simulink model "PSB3_0"  (R2021a)
settings: Solver=VariableStepAuto  StartTime=0.0  StopTime=3000  RelTol=1e-3
values from neighbouring files (symbols this model uses):
  n_channel = 1024    [PSB3_0_script.m]    (also in PSB_FPGAdesign8_script.m)
  parallel_factor = 4    [PSB3_0_script.m]    (also in PSB_FPGAdesign8_script.m)
libraries: xbsIndex_r4 x1051, xrbsSSR_Library x154, dspsrcs4 x26
(part 1 of 8)
settings Model: Creator=11037  LastModifiedBy=11037

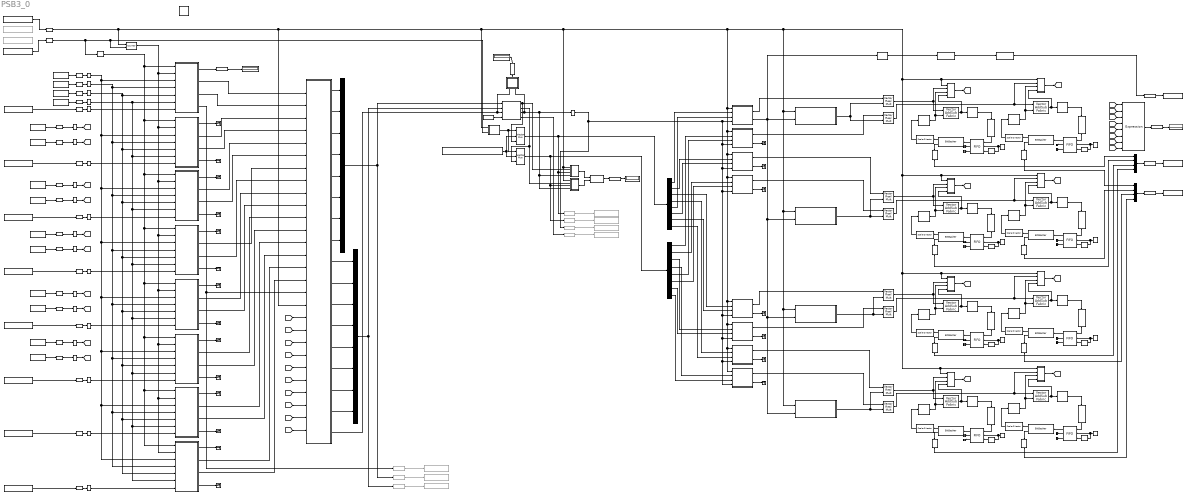
== system PSB3_0 ==
  note: Z^-(10+256)
  note: [zeros(1,50), ones(1,1024), 0]
  note: [zeros(1,50), ones(1,1024), 0]
  note: [zeros(1,50), ones(1,1024), 0]
  note: [zeros(1,50), ones(1,1024), 0]
  note: at t=0, the first samples out of vector FFT are NaN,
  note: With no integer bits at inputs and output, multiply will only saturate for the case of -1 x -1 = 1.
  " System Generator" : xbsIndex_r4/ System Generator  Tag=genX  xilinxfamily=zynquplusRFSOC  part=xczu28dr  speed=-2-e  package=ffvg1517  synthesis_tool=Vivado  clock_wrapper=Clock Enables  directory=C:/PSB3_0_NL  proj_type=Vivado  Synth_file=Vivado Synthesis Defaults  Impl_file=Vivado Implementation Defaults  testbench=off  simulink_period=1  sysclk_period=10  dcm_input_clock_period=10  incr_netlist=off  trim_vbits=Everywhere in SubSystem  dbl_ovrd=According to Block Masks  core_generation=According to Block Masks  run_coregen=off  deprecated_control=off  eval_field=0  block_type=sysgen
  0001_ : Subsystem
  Baseband_even_1 : Subsystem
  Baseband_even_2 : Subsystem
  Baseband_even_3 : Subsystem
  Baseband_even_4 : Subsystem
  Baseband_odd_1 : Subsystem
  Baseband_odd_2 : Subsystem
  Baseband_odd_3 : Subsystem
  Baseband_odd_4 : Subsystem
  BitBasher1 : xbsIndex_r4/BitBasher  bitexpr=|  display_expr=on  sr_1=a  arith_type1=Unsigned  bin_pt1=0  sr_2=b  arith_type2=Unsigned  bin_pt2=0  sr_3=3  arith_type3=Unsigned  bin_pt3=0  sr_4=4  arith_type4=Unsigned  bin_pt4=0  dbl_ovrd=off  block_type=bitbasher
      | a={16'b0, in[255:16]}
      | b={in[15:0]}
  BitBasher2 : xbsIndex_r4/BitBasher  bitexpr=|  display_expr=on  sr_1=a  arith_type1=Unsigned  bin_pt1=0  sr_2=b  arith_type2=Unsigned  bin_pt2=0  sr_3=3  arith_type3=Unsigned  bin_pt3=0  sr_4=4  arith_type4=Unsigned  bin_pt4=0  dbl_ovrd=off  block_type=bitbasher
      | a={16'b0, in[255:16]}
      | b={in[15:0]}
  BitBasher3 : xbsIndex_r4/BitBasher  bitexpr=|  display_expr=on  sr_1=a  arith_type1=Unsigned  bin_pt1=0  sr_2=b  arith_type2=Unsigned  bin_pt2=0  sr_3=3  arith_type3=Unsigned  bin_pt3=0  sr_4=4  arith_type4=Unsigned  bin_pt4=0  dbl_ovrd=off  block_type=bitbasher
      | a={16'b0, in[255:16]}
      | b={in[15:0]}
  BitBasher4 : xbsIndex_r4/BitBasher  bitexpr=|  display_expr=on  sr_1=a  arith_type1=Unsigned  bin_pt1=0  sr_2=b  arith_type2=Unsigned  bin_pt2=0  sr_3=3  arith_type3=Unsigned  bin_pt3=0  sr_4=4  arith_type4=Unsigned  bin_pt4=0  dbl_ovrd=off  block_type=bitbasher
      | a={16'b0, in[255:16]}
      | b={in[15:0]}
  BitBasher5 : xbsIndex_r4/BitBasher  bitexpr=|  display_expr=on  sr_1=a  arith_type1=Unsigned  bin_pt1=0  sr_2=b  arith_type2=Unsigned  bin_pt2=0  sr_3=3  arith_type3=Unsigned  bin_pt3=0  sr_4=4  arith_type4=Unsigned  bin_pt4=0  dbl_ovrd=off  block_type=bitbasher
      | a={16'b0, in[255:16]}
      | b={in[15:0]}
  BitBasher6 : xbsIndex_r4/BitBasher  bitexpr=|  display_expr=on  sr_1=a  arith_type1=Unsigned  bin_pt1=0  sr_2=b  arith_type2=Unsigned  bin_pt2=0  sr_3=3  arith_type3=Unsigned  bin_pt3=0  sr_4=4  arith_type4=Unsigned  bin_pt4=0  dbl_ovrd=off  block_type=bitbasher
      | a={16'b0, in[255:16]}
      | b={in[15:0]}
  BitBasher7 : xbsIndex_r4/BitBasher  bitexpr=|  display_expr=on  sr_1=a  arith_type1=Unsigned  bin_pt1=0  sr_2=b  arith_type2=Unsigned  bin_pt2=0  sr_3=3  arith_type3=Unsigned  bin_pt3=0  sr_4=4  arith_type4=Unsigned  bin_pt4=0  dbl_ovrd=off  block_type=bitbasher
      | a={16'b0, in[255:16]}
      | b={in[15:0]}
  BitBasher8 : xbsIndex_r4/BitBasher  bitexpr=|  display_expr=on  sr_1=a  arith_type1=Unsigned  bin_pt1=0  sr_2=b  arith_type2=Unsigned  bin_pt2=0  sr_3=3  arith_type3=Unsigned  bin_pt3=0  sr_4=4  arith_type4=Unsigned  bin_pt4=0  dbl_ovrd=off  block_type=bitbasher
      | a={16'b0, in[255:16]}
      | b={in[15:0]}
  CORDIC_delay_count_even_1 : Display
  Constant{1..6,14,16} (8 alike) : xbsIndex_r4/Constant  const=1  gui_display_data_type=Boolean  arith_type=Boolean  n_bits=16  bin_pt=14  preci_type=Single  exp_width=8  frac_width=24  explicit_period=on  period=1  equ=P=C  opselect=C  inp2=PCIN>>17  opr=+  inp1=P  carry=CIN  dbl_ovrd=off  block_type=constant
  Constant15 : xbsIndex_r4/Constant  const=2016  gui_display_data_type=Fixed-point  arith_type=Unsigned  n_bits=11  bin_pt=0  preci_type=Single  exp_width=8  frac_width=24  explicit_period=on  period=1  equ=P=C  opselect=C  inp2=PCIN>>17  opr=+  inp1=P  carry=CIN  dbl_ovrd=off  block_type=constant
  DPRAM_FIR_Coeffs_1 : Subsystem
  DPRAM_FIR_Coeffs_2 : Subsystem
  DPRAM_FIR_Coeffs_3 : Subsystem
  DPRAM_FIR_Coeffs_4 : Subsystem
  Delay{1..12,14,16,19,26,31,35,37..38,43..44,48..49} (24 alike) : xbsIndex_r4/Delay  rst=off  infoeditControl=Selection of Reset will increase slice count due to use of real FFs and instead of SRLs  en=off  latency=1  reg_retiming=off  dbl_ovrd=off  block_type=delay
  Delay{13,18,28..30,53,55..56} (8 alike) : xbsIndex_r4/Delay  rst=off  infoeditControl=Selection of Reset will increase slice count due to use of real FFs and instead of SRLs  en=off  latency=1024/parallel_factor-2-1  reg_retiming=off  dbl_ovrd=off  block_type=delay
  Delay15 : xbsIndex_r4/Delay  rst=off  infoeditControl=Selection of Reset will increase slice count due to use of real FFs and instead of SRLs  en=off  latency=2  reg_retiming=off  dbl_ovrd=off  block_type=delay
  Delay17 : xbsIndex_r4/Delay  rst=off  infoeditControl=Selection of Reset will increase slice count due to use of real FFs and instead of SRLs  en=off  latency=5  reg_retiming=off  dbl_ovrd=off  block_type=delay
  Delay54 : xbsIndex_r4/Delay  rst=off  infoeditControl=Selection of Reset will increase slice count due to use of real FFs and instead of SRLs  en=off  latency=1024/parallel_factor  reg_retiming=off  dbl_ovrd=off  block_type=delay
  Delay_duration : Display
  Demux : Demux  Outputs=8
  Demux1 : Demux  Outputs=8
  Display ov_add : Display
      settings: Format=decimal (Stored Integer)
  Expression : xbsIndex_r4/Expression  expression=a | b  align_bp=off  en=off  latency=1  precision=Full  arith_type=Unsigned  n_bits=1  bin_pt=0  dbl_ovrd=off  block_type=expr
  Expression1 : xbsIndex_r4/Expression  expression=a1 | b1 | c1 | d1 | a2 | b2 | c2 | d2  align_bp=off  en=off  latency=1  precision=Full  arith_type=Unsigned  n_bits=1  bin_pt=0  dbl_ovrd=off  block_type=expr
  FIFO{1..8} (8 alike) : xbsIndex_r4/FIFO  mem_type=Block RAM  performance_options=Standard_FIFO  embedded_registers=off  depth=1K  percent_nbits=1  rst=off  rst_latency=2  en=off  use_dcount=off  use_percent_full_port=off  use_almost_empty=off  almost_empty_thresh=2  use_almost_full=off  use_rd_rst_busy=off  use_wr_rst_busy=off  almost_full_thresh=14  explicit_period=off  dbl_ovrd=off  simulation_type=fast_sim  block_type=fifo
  Gin_TL_reset : xbsIndex_r4/Gateway In  gui_display_data_type=Boolean  arith_type=Boolean  n_bits=18  bin_pt=15  preci_type=Single  exp_width=8  frac_width=24  rows=1  columns=1  quantization="Round  (unbiased: +/- Inf)"  overflow=Flag as error  period=1  UseAsADC=off  ADCChannel='1'  interface=None  automatic_assignment=on  address_offset=hex2dec('00')  intf_name=''  intf_description=''  default_value=0  timing_constraint=None  locs_specified=off  LOCs={}  io_standard={}  inherit_from_input=off  hdl_port=on  dbl_ovrd=off  block_type=gatewayin
  Gin_TL_start : xbsIndex_r4/Gateway In  gui_display_data_type=Boolean  arith_type=Boolean  n_bits=18  bin_pt=15  preci_type=Single  exp_width=8  frac_width=24  rows=1  columns=1  quantization="Round  (unbiased: +/- Inf)"  overflow=Flag as error  period=1  UseAsADC=off  ADCChannel='1'  interface=None  automatic_assignment=on  address_offset=hex2dec('00')  intf_name=''  intf_description=''  default_value=0  timing_constraint=None  locs_specified=off  LOCs={}  io_standard={}  inherit_from_input=off  hdl_port=on  dbl_ovrd=off  block_type=gatewayin
  Gin_addr : xbsIndex_r4/Gateway In  gui_display_data_type=Fixed-point  arith_type=Unsigned  n_bits=10-2  bin_pt=0  preci_type=Single  exp_width=8  frac_width=24  rows=1  columns=1  quantization=Truncate  overflow=Flag as error  period=1  UseAsADC=off  ADCChannel='1'  interface=None  automatic_assignment=on  address_offset=hex2dec('00')  intf_name=''  intf_description=''  default_value=0  timing_constraint=None  locs_specified=off  LOCs={}  io_standard={}  inherit_from_input=off  hdl_port=on  dbl_ovrd=off  block_type=gatewayin
  Gin_dphi : xbsIndex_r4/Gateway In  gui_display_data_type=Fixed-point  arith_type=Unsigned  n_bits=16  bin_pt=0  preci_type=Single  exp_width=8  frac_width=24  rows=1  columns=1  quantization=Truncate  overflow=Flag as error  period=1  UseAsADC=off  ADCChannel='1'  interface=None  automatic_assignment=on  address_offset=hex2dec('00')  intf_name=''  intf_description=''  default_value=0  timing_constraint=None  locs_specified=off  LOCs={}  io_standard={}  inherit_from_input=off  hdl_port=on  dbl_ovrd=off  block_type=gatewayin
  Gin_init_im : xbsIndex_r4/Gateway In  gui_display_data_type=Fixed-point  arith_type="Signed  (2's comp)"  n_bits=18  bin_pt=16  preci_type=Single  exp_width=8  frac_width=24  rows=1  columns=1  quantization=Truncate  overflow=Flag as error  period=1  UseAsADC=off  ADCChannel='1'  interface=None  automatic_assignment=on  address_offset=hex2dec('00')  intf_name=''  intf_description=''  default_value=0  timing_constraint=None  locs_specified=off  LOCs={}  io_standard={}  inherit_from_input=off  hdl_port=on  dbl_ovrd=off  block_type=gatewayin
  Gin_init_re : xbsIndex_r4/Gateway In  gui_display_data_type=Fixed-point  arith_type="Signed  (2's comp)"  n_bits=18  bin_pt=16  preci_type=Single  exp_width=8  frac_width=24  rows=1  columns=1  quantization=Truncate  overflow=Flag as error  period=1  UseAsADC=off  ADCChannel='1'  interface=None  automatic_assignment=on  address_offset=hex2dec('00')  intf_name=''  intf_description=''  default_value=0  timing_constraint=None  locs_specified=off  LOCs={}  io_standard={}  inherit_from_input=off  hdl_port=on  dbl_ovrd=off  block_type=gatewayin
  Gin_we_even_{1..4} (4 alike) : xbsIndex_r4/Gateway In  gui_display_data_type=Boolean  arith_type=Boolean  n_bits=18  bin_pt=15  preci_type=Single  exp_width=8  frac_width=24  rows=1  columns=1  quantization="Round  (unbiased: +/- Inf)"  overflow=Flag as error  period=1  UseAsADC=off  ADCChannel='1'  interface=None  automatic_assignment=on  address_offset=hex2dec('00')  intf_name=''  intf_description=''  default_value=0  timing_constraint=None  locs_specified=off  LOCs={}  io_standard={}  inherit_from_input=off  hdl_port=on  dbl_ovrd=off  block_type=gatewayin
  Gin_we_odd_{1..4} (4 alike) : xbsIndex_r4/Gateway In  gui_display_data_type=Boolean  arith_type=Boolean  n_bits=18  bin_pt=15  preci_type=Single  exp_width=8  frac_width=24  rows=1  columns=1  quantization="Round  (unbiased: +/- Inf)"  overflow=Flag as error  period=1  UseAsADC=off  ADCChannel='1'  interface=None  automatic_assignment=on  address_offset=hex2dec('00')  intf_name=''  intf_description=''  default_value=0  timing_constraint=None  locs_specified=off  LOCs={}  io_standard={}  inherit_from_input=off  hdl_port=on  dbl_ovrd=off  block_type=gatewayin
  Gout_CORDIC_delay_even_1 : xbsIndex_r4/Gateway Out  inherit_from_input=on  hdl_port=on  rows=1  columns=1  UseAsDAC=off  DACChannel='1'  interface=None  automatic_assignment=on  address_offset=hex2dec('00')  intf_name=''  intf_description=''  timing_constraint=None  locs_specified=off  LOCs={}  io_standard={}  block_type=gatewayout
  Gout_CORDIC_im : xrbsSSR_Library/Vector Real Gateway Out  Commented=on  inherit_from_input=off  hdl_port=on  rows=1  columns=1  UseAsDAC=off  DACChannel='1'  interface=None  automatic_assignment=on  address_offset=hex2dec('00')  intf_name=''  intf_description=''  timing_constraint=None  locs_specified=off  LOCs={}  io_standard={}  block_type=realgatewayout_ssr  sg_ssr=8  sg_ssr_prev=8  sg_ssr_name=vect_real_gwayout
      settings: SourceProductName=Xilinx SSR Blockset  infoedit=The Vector Real Gateway out block converts Xilinx fixed-point or floating-point type vector inputs into vector ouputs of type Simulink integer, single, double, or fixed-point.<br><br>Hardware notes: In hardware these blocks become top level output ports or are discarded, depending on how they are configured.
  Gout_CORDIC_re : xrbsSSR_Library/Vector Real Gateway Out  Commented=on  inherit_from_input=on  hdl_port=on  rows=1  columns=1  UseAsDAC=off  DACChannel='1'  interface=None  automatic_assignment=on  address_offset=hex2dec('00')  intf_name=''  intf_description=''  timing_constraint=None  locs_specified=off  LOCs={}  io_standard={}  block_type=realgatewayout_ssr  sg_ssr=8  sg_ssr_prev=8  sg_ssr_name=vect_real_gwayout
      settings: SourceProductName=Xilinx SSR Blockset  infoedit=The Vector Real Gateway out block converts Xilinx fixed-point or floating-point type vector inputs into vector ouputs of type Simulink integer, single, double, or fixed-point.<br><br>Hardware notes: In hardware these blocks become top level output ports or are discarded, depending on how they are configured.
  Gout_CORDIC_tvalid : xbsIndex_r4/Gateway Out  Commented=on  inherit_from_input=on  hdl_port=on  rows=1  columns=1  UseAsDAC=off  DACChannel='1'  interface=None  automatic_assignment=on  address_offset=hex2dec('00')  intf_name=''  intf_description=''  timing_constraint=None  locs_specified=off  LOCs={}  io_standard={}  block_type=gatewayout
  Gout_PSB_im : xrbsSSR_Library/Vector Real Gateway Out  inherit_from_input=on  hdl_port=on  rows=1  columns=1  UseAsDAC=off  DACChannel='1'  interface=None  automatic_assignment=on  address_offset=hex2dec('00')  intf_name=''  intf_description=''  timing_constraint=None  locs_specified=off  LOCs={}  io_standard={}  block_type=realgatewayout_ssr  sg_ssr=4  sg_ssr_prev=4  sg_ssr_name=vect_real_gwayout
      settings: SourceProductName=Xilinx SSR Blockset  infoedit=The Vector Real Gateway out block converts Xilinx fixed-point or floating-point type vector inputs into vector ouputs of type Simulink integer, single, double, or fixed-point.<br><br>Hardware notes: In hardware these blocks become top level output ports or are discarded, depending on how they are configured.
  Gout_PSB_re : xrbsSSR_Library/Vector Real Gateway Out  inherit_from_input=on  hdl_port=on  rows=1  columns=1  UseAsDAC=off  DACChannel='1'  interface=None  automatic_assignment=on  address_offset=hex2dec('00')  intf_name=''  intf_description=''  timing_constraint=None  locs_specified=off  LOCs={}  io_standard={}  block_type=realgatewayout_ssr  sg_ssr=4  sg_ssr_prev=4  sg_ssr_name=vect_real_gwayout
      settings: SourceProductName=Xilinx SSR Blockset  infoedit=The Vector Real Gateway out block converts Xilinx fixed-point or floating-point type vector inputs into vector ouputs of type Simulink integer, single, double, or fixed-point.<br><br>Hardware notes: In hardware these blocks become top level output ports or are discarded, depending on how they are configured.
  Gout_PSB_tvalid : xbsIndex_r4/Gateway Out  inherit_from_input=on  hdl_port=on  rows=1  columns=1  UseAsDAC=off  DACChannel='1'  interface=None  automatic_assignment=on  address_offset=hex2dec('00')  intf_name=''  intf_description=''  timing_constraint=None  locs_specified=off  LOCs={}  io_standard={}  block_type=gatewayout
  Gout_delay_iFFT : xbsIndex_r4/Gateway Out  inherit_from_input=on  hdl_port=on  rows=1  columns=1  UseAsDAC=off  DACChannel='1'  interface=None  automatic_assignment=on  address_offset=hex2dec('00')  intf_name=''  intf_description=''  timing_constraint=None  locs_specified=off  LOCs={}  io_standard={}  block_type=gatewayout
  Gout_ov_IFFT : xbsIndex_r4/Gateway Out  inherit_from_input=on  hdl_port=on  rows=1  columns=1  UseAsDAC=off  DACChannel='1'  interface=None  automatic_assignment=on  address_offset=hex2dec('00')  intf_name=''  intf_description=''  timing_constraint=None  locs_specified=off  LOCs={}  io_standard={}  block_type=gatewayout
  Gout_ov_add : xbsIndex_r4/Gateway Out  inherit_from_input=on  hdl_port=on  rows=1  columns=1  UseAsDAC=off  DACChannel='1'  interface=None  automatic_assignment=on  address_offset=hex2dec('00')  intf_name=''  intf_description=''  timing_constraint=None  locs_specified=off  LOCs={}  io_standard={}  block_type=gatewayout
  Gout_vIFFT_im : xrbsSSR_Library/Vector Real Gateway Out  Commented=on  inherit_from_input=off  hdl_port=on  rows=1  columns=1  UseAsDAC=off  DACChannel='1'  interface=None  automatic_assignment=on  address_offset=hex2dec('00')  intf_name=''  intf_description=''  timing_constraint=None  locs_specified=off  LOCs={}  io_standard={}  block_type=realgatewayout_ssr  sg_ssr=8  sg_ssr_prev=8  sg_ssr_name=vect_real_gwayout
      settings: SourceProductName=Xilinx SSR Blockset  infoedit=The Vector Real Gateway out block converts Xilinx fixed-point or floating-point type vector inputs into vector ouputs of type Simulink integer, single, double, or fixed-point.<br><br>Hardware notes: In hardware these blocks become top level output ports or are discarded, depending on how they are configured.
  Gout_vIFFT_re : xrbsSSR_Library/Vector Real Gateway Out  Commented=on  inherit_from_input=off  hdl_port=on  rows=1  columns=1  UseAsDAC=off  DACChannel='1'  interface=None  automatic_assignment=on  address_offset=hex2dec('00')  intf_name=''  intf_description=''  timing_constraint=None  locs_specified=off  LOCs={}  io_standard={}  block_type=realgatewayout_ssr  sg_ssr=8  sg_ssr_prev=8  sg_ssr_name=vect_real_gwayout
      settings: SourceProductName=Xilinx SSR Blockset  infoedit=The Vector Real Gateway out block converts Xilinx fixed-point or floating-point type vector inputs into vector ouputs of type Simulink integer, single, double, or fixed-point.<br><br>Hardware notes: In hardware these blocks become top level output ports or are discarded, depending on how they are configured.
  Gout_vIFFT_scale : xbsIndex_r4/Gateway Out  Commented=on  inherit_from_input=on  hdl_port=on  rows=1  columns=1  UseAsDAC=off  DACChannel='1'  interface=None  automatic_assignment=on  address_offset=hex2dec('00')  intf_name=''  intf_description=''  timing_constraint=None  locs_specified=off  LOCs={}  io_standard={}  block_type=gatewayout
  Gout_vIFFT_tvalid : xbsIndex_r4/Gateway Out  Commented=on  inherit_from_input=off  hdl_port=on  rows=1  columns=1  UseAsDAC=off  DACChannel='1'  interface=None  automatic_assignment=on  address_offset=hex2dec('00')  intf_name=''  intf_description=''  timing_constraint=None  locs_specified=off  LOCs={}  io_standard={}  block_type=gatewayout
  Mux : Mux  Inputs=8
  Mux1 : Mux  Inputs=8
  Mux2 : Mux
  Mux3 : Mux
  Overflow Detector add_im_1 : Subsystem
  Overflow Detector add_im_2 : Subsystem
  Overflow Detector add_im_3 : Subsystem
  Overflow Detector add_im_4 : Subsystem
  Overflow Detector add_re_1 : Subsystem
  Overflow Detector add_re_2 : Subsystem
  Overflow Detector add_re_3 : Subsystem
  Overflow Detector add_re_4 : Subsystem
  RAM_dphi_addr : xbsIndex_r4/Counter  cnt_type=Free Running  cnt_to=Inf  operation=Up  start_count=0  cnt_by_val=1  arith_type=Unsigned  n_bits=10-2  bin_pt=0  load_pin=off  rst=on  en=on  explicit_period=on  period=1  use_behavioral_HDL=off  implementation=DSP48  dbl_ovrd=off  block_type=counter
  Reinterpret{,1..7} (8 alike) : xbsIndex_r4/Reinterpret  force_arith_type=on  arith_type="Signed  (2's comp)"  force_bin_pt=on  bin_pt=14  block_type=reinterpret
  Scalar to Vector{1..8} (8 alike) : xrbsSSR_Library/Scalar2Vector  Width=16  sg_ssr=16  sg_ssr_prev=16  sg_ssr_name=vect_Scalar2Vector  block_type=scalar2vector_ssr
      settings: SourceProductName=Xilinx SSR Blockset
  TL_reset : dspsrcs4/Signal From Workspace  Commented=on  X="[zeros(1,1000), ones(1,3000),  0]"  Ts=1  nsamps=1  OutputAfterFinalValue=Holding final value  ignoreOrWarnInputAndFrameLengths=on  OutputFrames=off
  TL_reset1 : dspsrcs4/Signal From Workspace  X=0  Ts=1  nsamps=1  OutputAfterFinalValue=Holding final value  ignoreOrWarnInputAndFrameLengths=on  OutputFrames=off
  TL_start : dspsrcs4/Signal From Workspace  Commented=on  X=[ones(1,1000), zeros(1,3000), 1]  Ts=1  nsamps=1  OutputAfterFinalValue=Holding final value  ignoreOrWarnInputAndFrameLengths=on  OutputFrames=off
  TL_start1 : dspsrcs4/Signal From Workspace  X=1  Ts=1  nsamps=1  OutputAfterFinalValue=Holding final value  ignoreOrWarnInputAndFrameLengths=on  OutputFrames=off
  TS_{0..7} (8 alike) : xbsIndex_r4/Gateway In  gui_display_data_type=Fixed-point  arith_type=Unsigned  n_bits=12  bin_pt=0  preci_type=Single  exp_width=8  frac_width=24  rows=1  columns=1  quantization=Truncate  overflow=Flag as error  period=1  UseAsADC=off  ADCChannel='1'  interface=None  automatic_assignment=on  address_offset=hex2dec('00')  intf_name=''  intf_description=''  default_value=0  timing_constraint=None  locs_specified=off  LOCs={}  io_standard={}  inherit_from_input=off  hdl_port=on  dbl_ovrd=off  block_type=gatewayin
  TS_A : xbsIndex_r4/Gateway In  gui_display_data_type=Fixed-point  arith_type=Unsigned  n_bits=8  bin_pt=0  preci_type=Single  exp_width=8  frac_width=24  rows=1  columns=1  quantization=Truncate  overflow=Flag as error  period=1  UseAsADC=off  ADCChannel='1'  interface=None  automatic_assignment=on  address_offset=hex2dec('00')  intf_name=''  intf_description=''  default_value=0  timing_constraint=None  locs_specified=off  LOCs={}  io_standard={}  inherit_from_input=off  hdl_port=on  dbl_ovrd=off  block_type=gatewayin
  TS_W : xbsIndex_r4/Gateway In  gui_display_data_type=Boolean  arith_type=Boolean  n_bits=18  bin_pt=15  preci_type=Single  exp_width=8  frac_width=24  rows=1  columns=1  quantization="Round  (unbiased: +/- Inf)"  overflow=Flag as error  period=1  UseAsADC=off  ADCChannel='1'  interface=None  automatic_assignment=on  address_offset=hex2dec('00')  intf_name=''  intf_description=''  default_value=0  timing_constraint=None  locs_specified=off  LOCs={}  io_standard={}  inherit_from_input=off  hdl_port=on  dbl_ovrd=off  block_type=gatewayin
  Terminator{,1..36} (37 alike) : Terminator
  To Workspace1 : ToWorkspace  Commented=on  VariableName=vIFFT_out_scale  SampleTime=1
  To Workspace10 : ToWorkspace  VariableName=PSB_out_im  SampleTime=1
  To Workspace2 : ToWorkspace  Commented=on  VariableName=vIFFT_out_re  SampleTime=1
  To Workspace3 : ToWorkspace  Commented=on  VariableName=vIFFT_out_im  SampleTime=1
  To Workspace4 : ToWorkspace  Commented=on  VariableName=CORDIC_out_re  SampleTime=1
  To Workspace5 : ToWorkspace  Commented=on  VariableName=vIFFT_out_tvalid  SampleTime=1
  To Workspace6 : ToWorkspace  VariableName=PSB_out_tvalid  SampleTime=1
  To Workspace7 : ToWorkspace  VariableName=PSB_out_re  SampleTime=1
  To Workspace8 : ToWorkspace  Commented=on  VariableName=CORDIC_out_im  SampleTime=1
  To Workspace9 : ToWorkspace  Commented=on  VariableName=CORDIC_out_tvalid  SampleTime=1
  ToneSelect : Subsystem
  Vector AddSub Fabric{,1..7} (8 alike) : xrbsSSR_Library/Vector AddSub Fabric  mode=Addition  use_carryin=off  use_carryout=off  en=off  sg_latency=2  precision=User Defined  arith_type="Signed  (2's comp)"  n_bits=16  bin_pt=14  quantization=Truncate  overflow=Flag as error  use_behavioral_HDL=off  hw_selection=DSP48  pipelined=off  dbl_ovrd=off  block_type=addsub_ssr  sg_ssr=16  sg_ssr_prev=16  sg_ssr_name=vect_addsubfab
      settings: SourceProductName=Xilinx SSR Blockset
  Vector Constant : xrbsSSR_Library/Vector Constant  const=[0.9 0.9 0.9 0.9 0.9 0.9 0.9 0.9]  gui_display_data_type=Fixed-point  arith_type=Signed (2's comp)  n_bits=16  bin_pt=15  preci_type=Single  exp_width=8  frac_width=24  explicit_period=on  period=1  sg_ssr=8  sg_ssr_prev=8  equ=P=C  opselect=C  inp2=PCIN>>17  opr=+  inp1=P  carry=CIN  dbl_ovrd=off  block_type=constant_ssr
      settings: SourceProductName=Xilinx SSR Blockset
  Vector Mux : xrbsSSR_Library/Vector Mux  inputs=2  inputs_prev=2  en=off  vectorize_en=off  vectorize_sel=off  sg_latency=1  precision=User Defined  arith_type="Signed  (2's comp)"  n_bits=16  bin_pt=15  quantization=Truncate  overflow=Saturate  dbl_ovrd=off  block_type=mux_ssr  sg_ssr=8  sg_ssr_prev=8  sg_ssr_name=vect_mux
      settings: SourceProductName=Xilinx SSR Blockset  infoedit=The Vector Multiplexer block supports Multiplexing feature for input of vector types.
  Vector Mux1 : xrbsSSR_Library/Vector Mux  inputs=2  inputs_prev=2  en=off  vectorize_en=off  vectorize_sel=off  sg_latency=1  precision=User Defined  arith_type="Signed  (2's comp)"  n_bits=16  bin_pt=15  quantization=Truncate  overflow=Saturate  dbl_ovrd=off  block_type=mux_ssr  sg_ssr=8  sg_ssr_prev=8  sg_ssr_name=vect_mux
      settings: SourceProductName=Xilinx SSR Blockset  infoedit=The Vector Multiplexer block supports Multiplexing feature for input of vector types.
  Vector Real Mult Im_{1..4} (4 alike) : xrbsSSR_Library/Vector Real Mult  sg_ssr=16  sg_ssr_prev=16  precision=User Defined  arith_type="Signed  (2's comp)"  n_bits=16  bin_pt=15  quantization=Truncate  overflow=Saturate  en=off  sg_latency=5  use_behavioral_HDL=off  opt=Speed  use_embedded=on  optimum_pipeline=off  pipeline=on  dbl_ovrd=off  use_rpm=on  placement_style=Triangular  block_type=realmult_ssr  sg_ssr_name=vect_realmult
      settings: SourceProductName=Xilinx SSR Blockset  infoedit=The Vector Real Multiplier block supports multiplicatoin feature for vector input types.<br><br>Hardware notes: To check for the optimum internal pipeline stages of the dedicated multiplier you must select 'Test for optimum pipelining'.<br><br>Optimization Goal: For implementation into device fabric(LUTs),the Speed and Area optimization will take effect only it its supported by IP for the particular device family. Otherwise, the results will be identical regardless of the selection.
  Vector Real Mult Re_{1..4} (4 alike) : xrbsSSR_Library/Vector Real Mult  sg_ssr=16  sg_ssr_prev=16  precision=User Defined  arith_type="Signed  (2's comp)"  n_bits=16  bin_pt=15  quantization=Truncate  overflow=Saturate  en=off  sg_latency=5  use_behavioral_HDL=off  opt=Speed  use_embedded=on  optimum_pipeline=off  pipeline=on  dbl_ovrd=off  use_rpm=on  placement_style=Triangular  block_type=realmult_ssr  sg_ssr_name=vect_realmult
      settings: SourceProductName=Xilinx SSR Blockset  infoedit=The Vector Real Multiplier block supports multiplicatoin feature for vector input types.<br><br>Hardware notes: To check for the optimum internal pipeline stages of the dedicated multiplier you must select 'Test for optimum pipelining'.<br><br>Optimization Goal: For implementation into device fabric(LUTs),the Speed and Area optimization will take effect only it its supported by IP for the particular device family. Otherwise, the results will be identical regardless of the selection.
  Vector Reinterpret{1..3,6,9..11,14} (8 alike) : xrbsSSR_Library/Vector Reinterpret  sg_ssr=16  sg_ssr_prev=16  force_arith_type=on  arith_type="Signed  (2's comp)"  force_bin_pt=on  bin_pt=14  block_type=reinterpret_ssr
      settings: SourceProductName=Xilinx SSR Blockset  infoedit="The Vector Reinterpret block Changes vector input signal type without altering the binary representation. You can change the signal between signed and unsigned, and relocate the binary point.<br><br>Hardware notes: In hardware this block costs nothing.<br><br>Example:  Suppose the input is 6 bits wide, signed, with 2 fractional bits, and the output is forced to unsigned with 0 fractional bits.  Then an input of -2.0 (1110.00 in binary 2's complement) becomes an output of 56 (111000 in binary)."
  Vector Reinterpret{4..5,7..8,12..13,15..16} (8 alike) : xrbsSSR_Library/Vector Reinterpret  sg_ssr=16  sg_ssr_prev=16  force_arith_type=on  arith_type=Unsigned  force_bin_pt=on  bin_pt=0  block_type=reinterpret_ssr
      settings: SourceProductName=Xilinx SSR Blockset  infoedit="The Vector Reinterpret block Changes vector input signal type without altering the binary representation. You can change the signal between signed and unsigned, and relocate the binary point.<br><br>Hardware notes: In hardware this block costs nothing.<br><br>Example:  Suppose the input is 6 bits wide, signed, with 2 fractional bits, and the output is forced to unsigned with 0 fractional bits.  Then an input of -2.0 (1110.00 in binary 2's complement) becomes an output of 56 (111000 in binary)."
  Vector to Scalar{,1..7} (8 alike) : xrbsSSR_Library/Vector2Scalar  sg_ssr=16  sg_ssr_prev=16  sg_ssr_name=vect_Vector2Scalar  block_type=vector2scalar_ssr
      settings: SourceProductName=Xilinx SSR Blockset
  delayCounter : Subsystem
  ov_IFFT Display : Display
      settings: Format=decimal (Stored Integer)
  ov_detector_IFFT_im : Subsystem
  ov_detector_IFFT_re : Subsystem
  reordering extending buffer imag_1 : Subsystem
  reordering extending buffer imag_2 : Subsystem
  reordering extending buffer imag_3 : Subsystem
  reordering extending buffer imag_4 : Subsystem
  reordering extending buffer real_1 : Subsystem
  reordering extending buffer real_2 : Subsystem
  reordering extending buffer real_3 : Subsystem
  reordering extending buffer real_4 : Subsystem
  test_TS_{0..7} (8 alike) : dspsrcs4/Signal From Workspace  X=0  Ts=1  nsamps=1  OutputAfterFinalValue=Setting to zero  ignoreOrWarnInputAndFrameLengths=on  OutputFrames=off
  test_TS_A : dspsrcs4/Signal From Workspace  X=0  Ts=1  nsamps=1  OutputAfterFinalValue=Setting to zero  ignoreOrWarnInputAndFrameLengths=on  OutputFrames=off
  test_TS_W : dspsrcs4/Signal From Workspace  X=0  Ts=1  nsamps=1  OutputAfterFinalValue=Setting to zero  ignoreOrWarnInputAndFrameLengths=on  OutputFrames=off
  vector IFFT : Subsystem
  w_addr : dspsrcs4/Signal From Workspace  X=[0:255]  Ts=1  nsamps=1  OutputAfterFinalValue=Setting to zero  ignoreOrWarnInputAndFrameLengths=on  OutputFrames=off
  w_dphi : dspsrcs4/Signal From Workspace  X=dphi_uint16_odd_4  Ts=1  nsamps=1  OutputAfterFinalValue=Setting to zero  ignoreOrWarnInputAndFrameLengths=on  OutputFrames=off
  w_init_im : dspsrcs4/Signal From Workspace  X=init_im_odd_4  Ts=1  nsamps=1  OutputAfterFinalValue=Setting to zero  ignoreOrWarnInputAndFrameLengths=on  OutputFrames=off
  w_init_re : dspsrcs4/Signal From Workspace  X=init_re_odd_4  Ts=1  nsamps=1  OutputAfterFinalValue=Setting to zero  ignoreOrWarnInputAndFrameLengths=on  OutputFrames=off
  we_even_{1..4} (4 alike) : dspsrcs4/Signal From Workspace  X=[0]  Ts=1  nsamps=1  OutputAfterFinalValue=Holding final value  ignoreOrWarnInputAndFrameLengths=on  OutputFrames=off
  we_odd_{1..4} (4 alike) : dspsrcs4/Signal From Workspace  X=[0]  Ts=1  nsamps=1  OutputAfterFinalValue=Holding final value  ignoreOrWarnInputAndFrameLengths=on  OutputFrames=off
  wires:
  Delay1/1 -> Baseband_even_1/7(we)
  Reinterpret2/1 -> Mux3/2
  Delay37/1 -> Baseband_even_1/6(dphi_even), Baseband_odd_1/6(dphi_odd), Baseband_even_2/6(dphi_even_2), Baseband_odd_2/6(dphi_odd_2), Baseband_even_3/6(dphi_even), Baseband_odd_3/6(dphi_odd), Baseband_even_4/6(dphi_even_2), Baseband_odd_4/6(dphi_odd_2)
  Constant16/1 -> Delay18/1, FIFO3/2
  Vector Real Mult Re_3/1 -> Overflow Detector add_re_3/2(A), Vector AddSub Fabric4/1
  reordering extending buffer real_4/2(out_tvalid) -> Terminator28/1
  Baseband_odd_3/4(out_tvalid) -> Terminator10/1
  0001_/1(out) -> Vector Mux1/1, Vector Mux/1
  Gout_vIFFT_tvalid/1 -> To Workspace5/1  "op_valid"
  we_odd_2/1 -> Gin_we_odd_2/1  "we"
  Reinterpret5/1 -> Mux2/4
  w_init_re/1 -> Gin_init_re/1
  Gin_TL_reset/1 -> ToneSelect/18(rst), ov_detector_IFFT_im/1(rst), ov_detector_IFFT_re/1(rst), reordering extending buffer imag_1/1(in_reset), reordering extending buffer real_2/1(in_reset), reordering extending buffer real_3/1(in_reset), reordering extending buffer real_4/1(in_reset), reordering extending buffer imag_4/1(in_reset), reordering extending buffer imag_3/1(in_reset), reordering extending buffer imag_2/1(in_reset), reordering extending buffer real_1/1(in_reset), Overflow Detector add_im_1/1(rst), Overflow Detector add_re_1/1(rst), Overflow Detector add_re_3/1(rst), Overflow Detector add_im_3/1(rst), Overflow Detector add_im_4/1(rst), Overflow Detector add_re_4/1(rst), Overflow Detector add_im_2/1(rst), Overflow Detector add_re_2/1(rst), DPRAM_FIR_Coeffs_1/1(In_rst), DPRAM_FIR_Coeffs_2/1(In_rst), DPRAM_FIR_Coeffs_3/1(In_rst), DPRAM_FIR_Coeffs_4/1(In_rst), 0001_/1(rst), RAM_dphi_addr/1
  FIFO4/1 -> BitBasher4/1
  Delay53/1 -> FIFO7/3
  FIFO1/1 -> BitBasher3/1
  Baseband_odd_2/4(out_tvalid) -> Terminator9/1
  BitBasher7/2 -> Reinterpret5/1
  Vector Reinterpret2/1 -> Overflow Detector add_re_1/3(B), Vector AddSub Fabric/2
  FIFO2/2 -> Terminator18/1
  Gout_vIFFT_scale/1 -> To Workspace1/1  "op_scale"
  Vector AddSub Fabric2/1 -> Overflow Detector add_re_2/4(S), Vector Reinterpret7/1
  Delay35/1 -> Baseband_even_1/5(init_re_even), Baseband_odd_1/5(init_re_odd), Baseband_even_2/5(init_re_even_2), Baseband_odd_2/5(init_re_odd_2), Baseband_even_3/5(init_re_even), Baseband_odd_3/5(init_re_odd), Baseband_even_4/5(init_re_even_2), Baseband_odd_4/5(init_re_odd_2)
  Delay38/1 -> Baseband_even_2/3(addr_w), Baseband_odd_2/3(addr_w), Baseband_even_3/3(addr_w), Baseband_odd_3/3(addr_w), Baseband_odd_4/3(addr_w), Baseband_even_4/3(addr_w), Baseband_odd_1/3(addr_w), Baseband_even_1/3(addr_w)
  Constant15/1 -> vector IFFT/4(SI)
  Vector to Scalar1/1 -> FIFO3/1
  Vector AddSub Fabric3/1 -> Overflow Detector add_im_2/4(S), Vector Reinterpret8/1
  FIFO2/3 -> Terminator21/1
  Baseband_odd_1/4(out_tvalid) -> Terminator7/1
  Vector to Scalar3/1 -> FIFO4/1
  Demux/8 -> reordering extending buffer real_4/3(input2)
  Baseband_odd_2/1(delay_count) -> Terminator34/1
  reordering extending buffer real_1/2(out_tvalid) -> DPRAM_FIR_Coeffs_3/2(In_en), DPRAM_FIR_Coeffs_4/2(In_en), DPRAM_FIR_Coeffs_2/2(In_en), DPRAM_FIR_Coeffs_1/2(In_en), Delay15/1
  Delay48/1 -> Baseband_odd_3/7(we)
  Vector Reinterpret10/1 -> Overflow Detector add_re_3/3(B), Vector AddSub Fabric4/2
  FIFO5/3 -> Terminator20/1
  Demux1/4 -> reordering extending buffer imag_4/2(input1)
  Gin_we_odd_2/1 -> Delay26/1
  Scalar to Vector6/1 -> Vector Reinterpret11/1
  Gin_addr/1 -> Delay38/1
  BitBasher4/2 -> Reinterpret2/1
  FIFO8/2 -> Terminator16/1
  Scalar to Vector7/1 -> Vector Reinterpret9/1
  Mux/1 -> vector IFFT/1(I.RE), Gout_CORDIC_re/1
  Gin_we_even_2/1 -> Delay8/1
  Vector Reinterpret16/1 -> Vector to Scalar7/1
  w_dphi/1 -> Gin_dphi/1
  Vector to Scalar7/1 -> FIFO8/1
  Constant3/1 -> Delay13/1, FIFO5/2
  Vector AddSub Fabric4/1 -> Overflow Detector add_re_3/4(S), Vector Reinterpret12/1
  Vector Reinterpret14/1 -> Overflow Detector add_im_4/3(B), Vector AddSub Fabric7/2
  we_odd_4/1 -> Gin_we_odd_4/1  "we"
  Vector Real Mult Im_3/1 -> Overflow Detector add_im_3/2(A), Vector AddSub Fabric5/1
  we_even_2/1 -> Gin_we_even_2/1  "we"
  TL_start1/1 -> Gin_TL_start/1  "TL_start"
  BitBasher7/1 -> Scalar to Vector7/1
  reordering extending buffer imag_1/1(vec_output) -> Vector Real Mult Im_1/1
  vector IFFT/4(SO) -> Gout_vIFFT_scale/1
  Vector to Scalar/1 -> FIFO2/1
  FIFO4/2 -> Terminator23/1
  BitBasher5/1 -> Scalar to Vector5/1
  Reinterpret4/1 -> Mux2/3
  Vector Real Mult Im_4/1 -> Overflow Detector add_im_4/2(A), Vector AddSub Fabric7/1
  Gin_we_odd_1/1 -> Delay6/1
  Reinterpret/1 -> Mux2/1
  Baseband_even_4/4(out_tvalid) -> Terminator11/1
  vector IFFT/3(VO) -> delayCounter/2(edge2), ov_detector_IFFT_im/4(en), ov_detector_IFFT_re/4(en), Delay19/1  "en"
  Delay19/1 -> reordering extending buffer imag_2/4(in_tvalid), reordering extending buffer real_3/4(in_tvalid), reordering extending buffer imag_4/4(in_tvalid), reordering extending buffer real_4/4(in_tvalid), reordering extending buffer imag_3/4(in_tvalid), reordering extending buffer real_2/4(in_tvalid), reordering extending buffer imag_1/4(in_tvalid), reordering extending buffer real_1/4(in_tvalid), Gout_vIFFT_tvalid/1
  FIFO6/2 -> Terminator3/1
  Gout_delay_iFFT/1 -> Delay_duration/1
  FIFO6/1 -> BitBasher5/1
  we_even_4/1 -> Gin_we_even_4/1  "we"
  Gout_PSB_tvalid/1 -> To Workspace6/1
  FIFO3/1 -> BitBasher2/1
  vector IFFT/1(O.RE) -> ov_detector_IFFT_re/2(A), Vector Mux/3  "A"
  Vector Reinterpret4/1 -> Vector to Scalar/1
  FIFO5/1 -> BitBasher7/1
  Delay28/1 -> FIFO2/3
  BitBasher4/1 -> Scalar to Vector4/1
  Vector AddSub Fabric1/1 -> Overflow Detector add_im_1/4(S), Vector Reinterpret5/1
  Vector AddSub Fabric6/1 -> Overflow Detector add_re_4/4(S), Vector Reinterpret15/1
  Vector Reinterpret12/1 -> Vector to Scalar4/1
  Baseband_even_2/4(out_tvalid) -> Terminator8/1
  FIFO7/2 -> Terminator29/1
  FIFO1/2 -> Terminator25/1
  Vector Reinterpret15/1 -> Vector to Scalar6/1
  Scalar to Vector1/1 -> Vector Reinterpret2/1
  Demux/1 -> reordering extending buffer real_1/2(input1)
  Gout_CORDIC_im/1 -> To Workspace8/1  "CORDIC_out_im"
  FIFO3/3 -> Terminator14/1
  Demux1/1 -> reordering extending buffer imag_1/2(input1)
  w_addr/1 -> Gin_addr/1
  reordering extending buffer imag_3/2(out_tvalid) -> Terminator27/1
  Demux1/8 -> reordering extending buffer imag_4/3(input2)
  Vector Reinterpret6/1 -> Overflow Detector add_im_2/3(B), Vector AddSub Fabric3/2
  w_init_im/1 -> Gin_init_im/1
  Vector Real Mult Im_1/1 -> Overflow Detector add_im_1/2(A), Vector AddSub Fabric1/1
  Vector Real Mult Re_2/1 -> Overflow Detector add_re_2/2(A), Vector AddSub Fabric2/1
  Mux3/1 -> Gout_PSB_im/1
  Baseband_even_3/1(delay_count) -> Terminator33/1
  reordering extending buffer imag_4/2(out_tvalid) -> Terminator4/1
  Vector Reinterpret9/1 -> Overflow Detector add_re_4/3(B), Vector AddSub Fabric6/2
  FIFO5/2 -> Terminator19/1
  FIFO4/3 -> Terminator24/1
  ov_detector_IFFT_im/1(ov) -> Expression/2
  Constant4/1 -> Delay55/1, FIFO6/2
  Overflow Detector add_im_3/1(ov) -> [c2]
  Overflow Detector add_re_3/1(ov) -> [c1]
  Baseband_even_2/1(delay_count) -> Terminator35/1
  reordering extending buffer imag_1/2(out_tvalid) -> Terminator/1
  Overflow Detector add_im_2/1(ov) -> [b2]
  Demux1/2 -> reordering extending buffer imag_2/2(input1)
  Vector AddSub Fabric/1 -> Overflow Detector add_re_1/4(S), Vector Reinterpret4/1
  Vector Reinterpret3/1 -> Overflow Detector add_im_1/3(B), Vector AddSub Fabric1/2
  Constant14/1 -> Delay28/1, FIFO2/2
  Overflow Detector add_im_4/1(ov) -> [d2]
  Constant2/1 -> Delay29/1, FIFO4/2
  ov_detector_IFFT_re/1(ov) -> Expression/1  "ov"
  Baseband_odd_4/4(out_tvalid) -> Terminator12/1
  Delay54/1 -> Gout_PSB_tvalid/1
  Baseband_even_1/4(out_tvalid) -> ToneSelect/17(In_tvalid), Gout_CORDIC_tvalid/1
  FIFO7/1 -> BitBasher6/1
  DPRAM_FIR_Coeffs_1/1(Out_FIR_Coeffs) -> Vector Real Mult Im_1/2, Vector Real Mult Re_1/2
  Constant1/1 -> Delay30/1, FIFO1/2
  FIFO3/2 -> Terminator13/1
  Gout_CORDIC_delay_even_1/1 -> CORDIC_delay_count_even_1/1
  Demux/3 -> reordering extending buffer real_3/2(input1)
  we_even_1/1 -> Gin_we_even_1/1  "we"
  Vector Mux1/1 -> Gout_vIFFT_im/1, ov_detector_IFFT_im/3(B), Demux1/1
  Gin_dphi/1 -> Delay37/1
  reordering extending buffer real_2/2(out_tvalid) -> Terminator1/1
  Vector AddSub Fabric5/1 -> Overflow Detector add_im_3/4(S), Vector Reinterpret13/1
  BitBasher3/1 -> Scalar to Vector3/1
  Demux1/5 -> reordering extending buffer imag_1/3(input2)
  Baseband_even_1/1(delay_count) -> Gout_CORDIC_delay_even_1/1
  BitBasher1/1 -> Scalar to Vector1/1
  FIFO2/1 -> BitBasher1/1
  Vector Real Mult Re_1/1 -> Overflow Detector add_re_1/2(A), Vector AddSub Fabric/1
  vector IFFT/2(O.IM) -> ov_detector_IFFT_im/2(A), Vector Mux1/3
  we_odd_3/1 -> Gin_we_odd_3/1  "we"
  Gout_vIFFT_im/1 -> To Workspace3/1  "op_im"
  Mux2/1 -> Gout_PSB_re/1
  BitBasher2/1 -> Scalar to Vector2/1
  BitBasher8/1 -> Scalar to Vector8/1
  Delay49/1 -> Baseband_even_4/7(we)
  Vector Reinterpret11/1 -> Overflow Detector add_im_3/3(B), Vector AddSub Fabric5/2
  Gin_init_re/1 -> Delay35/1
  we_even_3/1 -> Gin_we_even_3/1  "we"
  reordering extending buffer imag_2/2(out_tvalid) -> Terminator6/1
  Vector Mux/1 -> Gout_vIFFT_re/1, ov_detector_IFFT_re/3(B), Demux/1  "B"
  Gout_PSB_re/1 -> To Workspace7/1
  Delay8/1 -> Baseband_even_2/7(we)
  Demux/7 -> reordering extending buffer real_3/3(input2)
  Vector Reinterpret5/1 -> Vector to Scalar1/1
  Vector Constant/1 -> Vector Mux1/2, Vector Mux/2
  reordering extending buffer real_3/1(vec_output) -> Vector Real Mult Re_3/1
  Delay18/1 -> FIFO3/3
  reordering extending buffer real_4/1(vec_output) -> Vector Real Mult Re_4/1
  reordering extending buffer real_1/1(vec_output) -> Vector Real Mult Re_1/1
  Delay31/1 -> Baseband_even_3/7(we)
  Gin_TL_start/1 -> 0001_/2(en), RAM_dphi_addr/2, Delay14/1
  Demux1/7 -> reordering extending buffer imag_3/3(input2)
  we_odd_1/1 -> Gin_we_odd_1/1  "we"
  Gin_we_odd_4/1 -> Delay43/1
  BitBasher1/2 -> Reinterpret/1
  Baseband_odd_3/1(delay_count) -> Terminator32/1
  FIFO1/3 -> Terminator26/1
  Mux1/1 -> vector IFFT/2(I.IM), Gout_CORDIC_im/1
  Gout_CORDIC_re/1 -> To Workspace4/1  "CORDIC_out_re"
  Gout_PSB_im/1 -> To Workspace10/1
  Reinterpret3/1 -> Mux3/1
  Scalar to Vector2/1 -> Vector Reinterpret3/1
  Scalar to Vector8/1 -> Vector Reinterpret14/1
  Gin_we_even_3/1 -> Delay31/1
  Vector to Scalar4/1 -> FIFO6/1
  BitBasher6/1 -> Scalar to Vector6/1
  [b2] -> Expression1/4
  reordering extending buffer real_3/2(out_tvalid) -> Terminator22/1
  [a2] -> Expression1/2
  Delay29/1 -> FIFO4/3
  FIFO8/1 -> BitBasher8/1
  Overflow Detector add_re_2/1(ov) -> [b1]
  Vector Real Mult Im_2/1 -> Overflow Detector add_im_2/2(A), Vector AddSub Fabric3/1
  Vector Reinterpret8/1 -> Vector to Scalar3/1
  Demux/2 -> reordering extending buffer real_2/2(input1)
  Overflow Detector add_im_1/1(ov) -> [a2]
  Delay26/1 -> Baseband_odd_2/7(we)
  Vector Reinterpret7/1 -> Vector to Scalar2/1
  BitBasher3/2 -> Reinterpret1/1
  Constant5/1 -> Delay53/1, FIFO7/2
  [d2] -> Expression1/8
  Delay56/1 -> FIFO8/3
  BitBasher2/2 -> Reinterpret3/1
  Gin_we_odd_3/1 -> Delay48/1
  Gin_we_even_4/1 -> Delay49/1
  Overflow Detector add_re_1/1(ov) -> [a1]
  Scalar to Vector5/1 -> Vector Reinterpret10/1
  Baseband_even_3/4(out_tvalid) -> Terminator15/1
  [d1] -> Expression1/7
  Reinterpret7/1 -> Mux3/3
  Gout_vIFFT_re/1 -> To Workspace2/1  "op_re"
  [c1] -> Expression1/5
  [c2] -> Expression1/6
  delayCounter/1(delay) -> Gout_delay_iFFT/1
  Delay15/1 -> Delay17/1
  Gin_init_im/1 -> Delay44/1
  Baseband_odd_1/1(delay_count) -> Terminator36/1
  BitBasher5/2 -> Reinterpret4/1
  Gout_ov_add/1 -> Display ov_add/1
  Delay30/1 -> FIFO1/3
  Demux/4 -> reordering extending buffer real_4/2(input1)
  Vector to Scalar5/1 -> FIFO7/1
  Gout_ov_IFFT/1 -> ov_IFFT Display/1
  FIFO6/3 -> Terminator5/1
  Expression1/1 -> Gout_ov_add/1
  RAM_dphi_addr/1 -> Baseband_even_2/2(addr_r), Baseband_even_3/2(addr_r), Baseband_odd_3/2(addr_r), Baseband_odd_4/2(addr_r), Baseband_even_4/2(addr_r), Baseband_odd_2/2(addr_r), Baseband_odd_1/2(addr_r), Baseband_even_1/2(addr_r)
  [b1] -> Expression1/3
  Vector Reinterpret13/1 -> Vector to Scalar5/1
  Expression/1 -> Gout_ov_IFFT/1
  Reinterpret6/1 -> Mux3/4
  Vector AddSub Fabric7/1 -> Overflow Detector add_im_4/4(S), Vector Reinterpret16/1
  Gout_CORDIC_tvalid/1 -> To Workspace9/1  "CORDIC_out_tvalid"
  Delay14/1 -> Baseband_even_2/1(in_tvalid), Baseband_even_3/1(in_tvalid), Baseband_odd_3/1(tvalid), Baseband_odd_4/1(tvalid), Baseband_even_4/1(in_tvalid), Baseband_odd_2/1(tvalid), Baseband_odd_1/1(tvalid), Baseband_even_1/1(in_tvalid)
  TL_reset1/1 -> Gin_TL_reset/1  "TL_reset"
  reordering extending buffer imag_4/1(vec_output) -> Vector Real Mult Im_4/1
  Baseband_even_4/1(delay_count) -> Terminator31/1
  Delay17/1 -> Delay54/1
  Delay6/1 -> Baseband_odd_1/7(we)
  reordering extending buffer real_2/1(vec_output) -> Vector Real Mult Re_2/1
  Scalar to Vector3/1 -> Vector Reinterpret1/1
  Baseband_odd_4/1(delay_count) -> Terminator30/1
  Demux1/6 -> reordering extending buffer imag_2/3(input2)
  Delay43/1 -> Baseband_odd_4/7(we)
  FIFO8/3 -> Terminator17/1
  FIFO7/3 -> Terminator2/1
  Demux1/3 -> reordering extending buffer imag_3/2(input1)
  Demux/5 -> reordering extending buffer real_1/3(input2)
  Vector Real Mult Re_4/1 -> Overflow Detector add_re_4/2(A), Vector AddSub Fabric6/1
  reordering extending buffer imag_2/1(vec_output) -> Vector Real Mult Im_2/1
  Delay44/1 -> Baseband_even_1/4(init_im_even), Baseband_odd_1/4(init_im_odd), Baseband_even_2/4(init_im_even_2), Baseband_odd_2/4(init_im_odd_2), Baseband_even_3/4(init_im_even), Baseband_odd_3/4(init_im_odd), Baseband_odd_4/4(init_im_odd_2), Baseband_even_4/4(init_im_even_2)
  BitBasher8/2 -> Reinterpret6/1
  Vector Reinterpret1/1 -> Overflow Detector add_re_2/3(B), Vector AddSub Fabric2/2
  reordering extending buffer imag_3/1(vec_output) -> Vector Real Mult Im_3/1
  Reinterpret1/1 -> Mux2/2
  Scalar to Vector4/1 -> Vector Reinterpret6/1
  DPRAM_FIR_Coeffs_3/1(Out_FIR_Coeffs) -> Vector Real Mult Re_3/2, Vector Real Mult Im_3/2
  [a1] -> Expression1/1
  Vector to Scalar6/1 -> FIFO5/1
  Delay13/1 -> FIFO5/3
  Gin_we_even_1/1 -> Delay1/1
  Constant6/1 -> Delay56/1, FIFO8/2
  DPRAM_FIR_Coeffs_2/1(Out_FIR_Coeffs) -> Vector Real Mult Im_2/2, Vector Real Mult Re_2/2
  Vector to Scalar2/1 -> FIFO1/1
  BitBasher6/2 -> Reinterpret7/1
  Demux/6 -> reordering extending buffer real_2/3(input2)
  DPRAM_FIR_Coeffs_4/1(Out_FIR_Coeffs) -> Vector Real Mult Im_4/2, Vector Real Mult Re_4/2
  Overflow Detector add_re_4/1(ov) -> [d1]
  Delay55/1 -> FIFO6/3
  ToneSelect/1(Out_even1_re) -> Mux/1
  ToneSelect/2(Out_odd1_re) -> Mux/2
  ToneSelect/3(Out_even2_re) -> Mux/3
  ToneSelect/4(Out_odd2_re) -> Mux/4
  ToneSelect/5(Out_even3_re) -> Mux/5
  ToneSelect/6(Out_odd3_re) -> Mux/6
  ToneSelect/7(Out_even4_re) -> Mux/7
  ToneSelect/8(Out_odd4_re) -> Mux/8
  ToneSelect/9(Out_even1_im) -> Mux1/1
  ToneSelect/10(Out_odd1_im) -> Mux1/2
  ToneSelect/11(Out_even2_im) -> Mux1/3
  ToneSelect/12(Out_odd2_im) -> Mux1/4
  ToneSelect/13(Out_even3_im) -> Mux1/5
  ToneSelect/14(Out_odd3_im) -> Mux1/6
  ToneSelect/15(Out_even4_im) -> Mux1/7
  ToneSelect/16(Out_odd4_im) -> Mux1/8
  ToneSelect/17(Out_tvalid) -> delayCounter/1(edge1), vector IFFT/3(VI)
  Baseband_even_1/2(out_im) -> ToneSelect/1(In_even1_im)
  Baseband_even_1/3(out_re) -> ToneSelect/2(In_even1_re)
  Baseband_odd_1/2(out_im) -> ToneSelect/3(In_odd1_im)
  Baseband_odd_1/3(out_re) -> ToneSelect/4(In_odd1_re)
  Baseband_even_2/2(out_im) -> ToneSelect/5(In_even2_im)
  Baseband_even_2/3(out_re) -> ToneSelect/6(In_even2_re)
  Baseband_odd_2/2(out_im) -> ToneSelect/7(In_odd2_im)
  Baseband_odd_2/3(out_re) -> ToneSelect/8(In_odd2_re)
  Baseband_even_3/2(out_im) -> ToneSelect/9(In_even3_im)
  Baseband_even_3/3(out_re) -> ToneSelect/10(In_even3_re)
  Baseband_odd_3/2(out_im) -> ToneSelect/11(In_odd3_im)
  Baseband_odd_3/3(out_re) -> ToneSelect/12(In_odd3_re)
  Baseband_even_4/2(out_im) -> ToneSelect/13(In_even4_im)
  Baseband_even_4/3(out_re) -> ToneSelect/14(In_even4_re)
  Baseband_odd_4/2(out_im) -> ToneSelect/15(In_odd4_im)
  Baseband_odd_4/3(out_re) -> ToneSelect/16(In_odd4_re)
  [TS_0] -> ToneSelect/19(data_0)
  [TS_1] -> ToneSelect/20(data_1)
  [TS_2] -> ToneSelect/21(data_2)
  [TS_3] -> ToneSelect/22(data_3)
  [TS_4] -> ToneSelect/23(data_4)
  [TS_5] -> ToneSelect/24(data_5)
  [TS_6] -> ToneSelect/25(data_6)
  [TS_7] -> ToneSelect/26(data_7)
  [TS_A] -> ToneSelect/27(w_addr)
  [TS_W] -> ToneSelect/28(we)
  Delay2/1 -> [TS_0]
  Delay3/1 -> [TS_1]
  TS_0/1 -> Delay2/1
  TS_1/1 -> Delay3/1
  test_TS_0/1 -> TS_0/1
  test_TS_1/1 -> TS_1/1
  TS_3/1 -> Delay5/1
  Delay5/1 -> [TS_3]
  test_TS_2/1 -> TS_2/1
  test_TS_3/1 -> TS_3/1
  Delay4/1 -> [TS_2]
  TS_2/1 -> Delay4/1
  TS_5/1 -> Delay9/1
  Delay9/1 -> [TS_5]
  test_TS_4/1 -> TS_4/1
  test_TS_5/1 -> TS_5/1
  Delay7/1 -> [TS_4]
  TS_4/1 -> Delay7/1
  TS_7/1 -> Delay11/1
  Delay11/1 -> [TS_7]
  test_TS_6/1 -> TS_6/1
  test_TS_7/1 -> TS_7/1
  Delay10/1 -> [TS_6]
  TS_6/1 -> Delay10/1
  TS_W/1 -> Delay16/1
  Delay16/1 -> [TS_W]
  test_TS_A/1 -> TS_A/1
  test_TS_W/1 -> TS_W/1
  Delay12/1 -> [TS_A]
  TS_A/1 -> Delay12/1

== system PSB3_0/0001_ ==
  rst : Inport
  en : Inport  Port=2
  Constant17 : xbsIndex_r4/Constant  const=3  gui_display_data_type=Fixed-point  arith_type=Unsigned  n_bits=2  bin_pt=0  preci_type=Single  exp_width=8  frac_width=24  explicit_period=on  period=1  equ=P=C  opselect=C  inp2=PCIN>>17  opr=+  inp1=P  carry=CIN  dbl_ovrd=off  block_type=constant
  Counter : xbsIndex_r4/Counter  cnt_type=Free Running  cnt_to=3  operation=Up  start_count=0  cnt_by_val=1  arith_type=Unsigned  n_bits=2  bin_pt=0  load_pin=off  rst=on  en=on  explicit_period=on  period=1  use_behavioral_HDL=off  implementation=Fabric  dbl_ovrd=off  block_type=counter
  Register : xbsIndex_r4/Register  init=0  rst=on  en=on  dbl_ovrd=off  block_type=register
  Relational : xbsIndex_r4/Relational  mode=a>=b  op_type=Bool  en=off  latency=1  dbl_ovrd=off  block_type=relational
  const : xbsIndex_r4/Constant  const=1  gui_display_data_type=Boolean  arith_type=Boolean  n_bits=18  bin_pt=16  preci_type=Single  exp_width=8  frac_width=24  explicit_period=on  period=1  equ=P=C  opselect=C  inp2=PCIN>>17  opr=+  inp1=P  carry=CIN  dbl_ovrd=off  block_type=constant
  out : Outport
  wires:
  Counter/1 -> Relational/1
  const/1 -> Register/1
  rst/1 -> Counter/1, Register/2
  Register/1 -> out/1
  Constant17/1 -> Relational/2
  Relational/1 -> Register/3
  en/1 -> Counter/2
